simulink model "RotaryFlexLink_Workspace"  (R2021a)
settings: Solver=ode4  StartTime=0.0  StopTime=inf  FixedStep=0.001  RelTol=1e-3  EnableMultiTasking=on
model workspace (MAT data in the model file):
  Fc_est = 0.030885
  Jeq_est = 0.00174469
  Jl = 0.0038056
  Ll = 0.4191
  Rm_est = 3.11197
  beq_est = 0.0024798
  bl_est = 0.005635968
  km_est = 0.00744539
  ks_est = 1.3933
  kt_est = 0.00744539
  ml = 0.065
libraries: quarc_library x4, simulink x1
settings Model: SimulationMode=external  ExtModeTrigDuration=10000  Creator=MLevis  LastModifiedBy=pmartin
settings SolverCC: AlgebraicLoopSolver=TrustRegion  PositivePriorityOrder=on
settings DataIOCC: ReturnWorkspaceOutputs=off
settings DebuggingCC: SFMachineParentedDataDiag=warning  ArithmeticOperatorsInVariantConditions=warning
settings SFSimCC: SimUseLocalCustomCode=off  CustomCodeUndefinedFunction=UseInterfaceOnly
settings RTWCC: Description=QUARC Win64 Target Using Toolchain  SystemTargetFile=quarc_win64.tlc  TemplateMakefile=quarc_default_tmf  RTWUseLocalCustomCode=off  Toolchain=QUARC win64 | nmake (64-bit Windows)  BuildConfiguration=Faster Runs
settings CodeAppCC: StateflowObjectComments=on
settings STFCustomTargetCC: TargetLangStandard=C99 (ISO)  ConcurrentExecutionCompliant=on  SystemTargetFile=quarc_win64.tlc
settings GRTTargetCC: ParMdlRefBuildCompliant=off  CompOptLevelCompliant=off  CombineOutputUpdateFcns=off  MatFileLogging=off  CPPClassGenCompliant=off  GRTInterface=on  ExtMode=on  ExtModeMexFile=quarc_comm
settings ConfigComp: CovMetricSettings=dswe

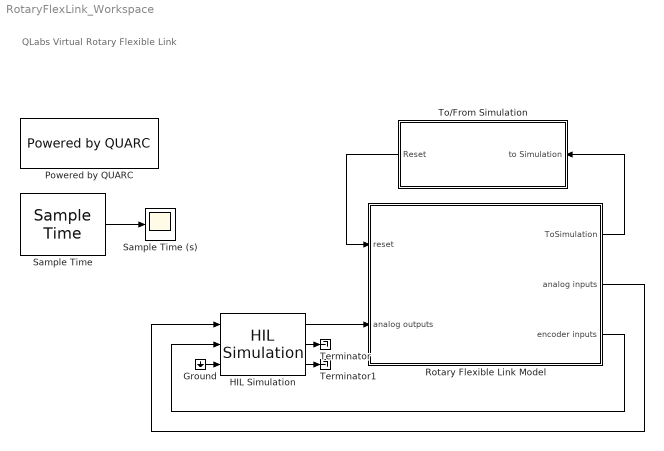
== system RotaryFlexLink_Workspace ==
  note: QLabs Virtual Rotary Flexible Link
  Ground : Ground
  HIL Simulation : quarc_library/Data Acquisition/Generic/Configuration/HIL Simulation  uri=tcpip://localhost:18941  board_type=q8_usb  board_id=0  sample_time=qc_get_step_size  active=on  num_clocks=1  num_interrupts=0  num_analog_inputs=8  num_analog_outputs=8  initial_analog=[]  num_digital_io=0  num_digital_inputs=8  num_digital_outputs=8  initial_digital=[]  num_encoder_inputs=8  num_pwm_outputs=8  initial_pwm=[]  other_inputs=[]  other_outputs=[]  initial_other=[]  integer_properties=[]  double_properties=[]  string_properties=[]
      settings: SourceProductName=QUARC Targets
  Powered by QUARC : quarc_library/Logos/Powered by QUARC
  Rotary Flexible Link Model : Subsystem
  Sample Time : quarc_library/Sources/Time/Sample Time  Priority=-99  sample_time=qc_get_step_size
  Sample Time (s) : Scope
  Terminator : Terminator
  Terminator1 : Terminator
  To/From Simulation : Subsystem
  wires:
  Rotary Flexible Link Model/3(encoder inputs) -> HIL Simulation/2
  Rotary Flexible Link Model/2(analog inputs) -> HIL Simulation/1
  HIL Simulation/1 -> Rotary Flexible Link Model/2(analog outputs)
  Sample Time/1 -> Sample Time (s)/1
  Rotary Flexible Link Model/1(ToSimulation) -> To/From Simulation/1(to Simulation)
  To/From Simulation/1(Reset) -> Rotary Flexible Link Model/1(reset)
  Ground/1 -> HIL Simulation/3
  HIL Simulation/2 -> Terminator/1
  HIL Simulation/3 -> Terminator1/1

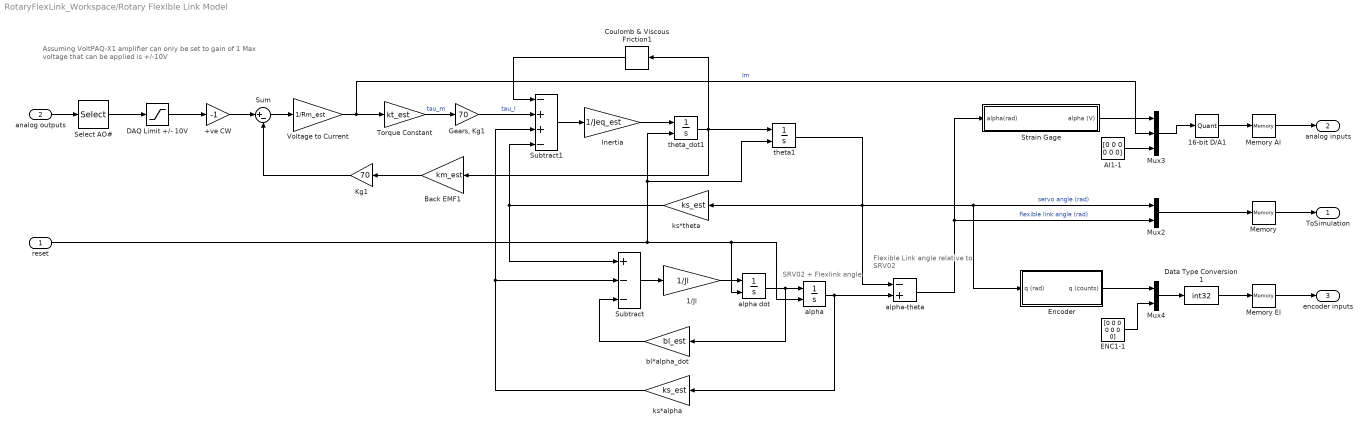
== system RotaryFlexLink_Workspace/Rotary Flexible Link Model ==
  note: Flexible Link angle
      | relative to SRV02
  note: SRV02 + Flexlink angle
  note: Assuming VoltPAQ-X1 amplifier can only be set to gain of 1
      | Max voltage that can be applied is +/-10V
  reset : Inport
  analog outputs : Inport  Port=2
  +ve CW : Gain  Gain=-1
  1/Jl : Gain  Gain=1/Jl  SaturateOnIntegerOverflow=on  OutDataTypeStr=Inherit: Same as input  ParamDataTypeStr=Inherit: Same as input
  16-bit D/A1 : Quantizer  QuantizationInterval=1/2^16
  AI1-1 : Constant  Value=[0 0 0 0 0 0]
  Back EMF1 : Gain  Gain=km_est  SaturateOnIntegerOverflow=on  OutDataTypeStr=Inherit: Same as input  ParamDataTypeStr=Inherit: Same as input
  Coulomb & Viscous Friction1 : simulink/Discontinuities/Coulomb & Viscous Friction  offset=[Fc_est]  gain=beq_est
  DAQ Limit +/- 10V : Saturate  UpperLimit=10  LowerLimit=-10
  Data Type Conversion1 : DataTypeConversion  OutDataTypeStr=int32
  ENC1-1 : Constant  Value=[0 0 0 0 0 0 0]
  Encoder : Subsystem
  "Gears, Kg1" : Gain  Gain=70
  Inertia : Gain  Gain=1/Jeq_est  SaturateOnIntegerOverflow=on  OutDataTypeStr=Inherit: Same as input  ParamDataTypeStr=Inherit: Same as input
  Kg1 : Gain  Gain=70
  Memory : Memory  InitialCondition=[0 0]
  Memory AI : Memory  InitialCondition=[0 0 0 0 0 0 0 0]  InheritSampleTime=on
  Memory EI : Memory  InitialCondition=[0 0 0 0 0 0 0 0]  InheritSampleTime=on
  Mux2 : Mux  Inputs=2
  Mux3 : Mux  Inputs=3
  Mux4 : Mux  Inputs=2
  Select AO# : Selector  InputPortWidth=8  IndexOptions=Index vector (dialog)  Indices=[1]  OutputSizes=1
  Strain Gage : Subsystem
  Subtract : Sum  Inputs=+--
  Subtract1 : Sum  Inputs=-++-
  Sum : Sum  Inputs=|+-  InputSameDT=on  SaturateOnIntegerOverflow=on  OutDataTypeStr=Inherit: Same as first input
  Torque Constant : Gain  Gain=kt_est
  Voltage to Current : Gain  Gain=1/Rm_est  SaturateOnIntegerOverflow=on  OutDataTypeStr=Inherit: Same as input  ParamDataTypeStr=Inherit: Same as input
  alpha : Integrator  ExternalReset=rising
  alpha dot : Integrator  ExternalReset=rising
  alpha-theta : Sum  Inputs=-+
  bl*alpha_dot : Gain  Gain=bl_est
  ks*alpha : Gain  Gain=ks_est
  ks*theta : Gain  Gain=ks_est
  theta1 : Integrator  ExternalReset=rising
  theta_dot1 : Integrator  ExternalReset=rising
  ToSimulation : Outport  VectorParamsAs1DForOutWhenUnconnected=off
  analog inputs : Outport  Port=2  VectorParamsAs1DForOutWhenUnconnected=off
  encoder inputs : Outport  Port=3  VectorParamsAs1DForOutWhenUnconnected=off
  wires:
  Memory/1 -> ToSimulation/1
  reset/1 -> theta1/2, theta_dot1/2, alpha dot/2, alpha/2
  Mux2/1 -> Memory/1
  Coulomb & Viscous Friction1/1 -> Subtract1/1
  Inertia/1 -> theta_dot1/1
  Sum/1 -> Voltage to Current/1
  bl*alpha_dot/1 -> Subtract/3
  ks*alpha/1 -> Subtract/2, Subtract1/3
  theta1/1 -> ks*theta/1, alpha-theta/1, Encoder/1(q (rad)), Mux2/1  "servo angle (rad)"
  Voltage to Current/1 -> Mux3/2, Torque Constant/1  "Im"
  Torque Constant/1 -> "Gears, Kg1"/1  "tau_m"
  Subtract/1 -> 1/Jl/1
  1/Jl/1 -> alpha dot/1
  Kg1/1 -> Sum/2
  ks*theta/1 -> Subtract/1, Subtract1/4
  "Gears, Kg1"/1 -> Subtract1/2  "tau_l"
  alpha dot/1 -> bl*alpha_dot/1, alpha/1
  theta_dot1/1 -> Coulomb & Viscous Friction1/1, theta1/1, Back EMF1/1
  Subtract1/1 -> Inertia/1
  alpha-theta/1 -> Strain Gage/1(alpha(rad)), Mux2/2  "flexible link angle (rad)"
  Back EMF1/1 -> Kg1/1
  +ve CW/1 -> Sum/1
  alpha/1 -> alpha-theta/2, ks*alpha/1
  analog outputs/1 -> Select AO#/1
  Select AO#/1 -> DAQ Limit +/- 10V/1
  DAQ Limit +/- 10V/1 -> +ve CW/1
  Mux3/1 -> 16-bit D/A1/1
  Encoder/1(q (counts)) -> Mux4/1
  Memory EI/1 -> encoder inputs/1
  Data Type Conversion1/1 -> Memory EI/1
  16-bit D/A1/1 -> Memory AI/1
  Mux4/1 -> Data Type Conversion1/1
  ENC1-1/1 -> Mux4/2
  AI1-1/1 -> Mux3/3
  Memory AI/1 -> analog inputs/1
  Strain Gage/1(alpha (V)) -> Mux3/1

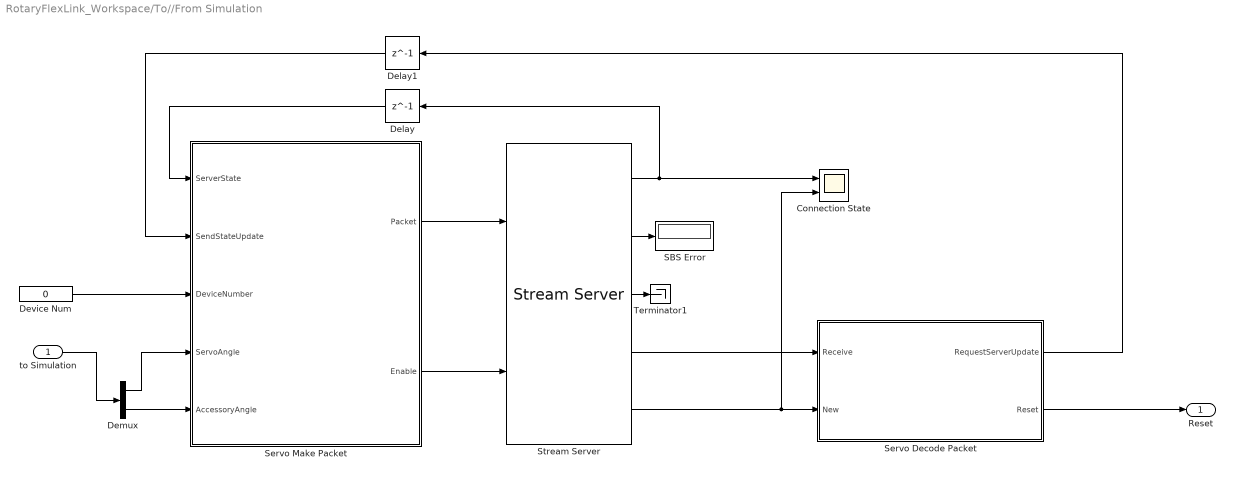
== system RotaryFlexLink_Workspace/To//From Simulation ==
  to Simulation : Inport
  "Connection State " : Scope  NumInputPorts=2
  Delay : Delay  DelayLength=1
  Delay1 : Delay  DelayLength=1
  Demux : Demux  Outputs=2
  Device Num : Constant  Value=0
  SBS Error : Display
  Servo Decode Packet : MATLAB Function  TreatAsAtomicUnit=on
  Servo Make Packet : MATLAB Function  TreatAsAtomicUnit=on
  Stream Server : quarc_library/Communications/Basic/Stream Server  uri_source=Specify via dialog (do not evaluate)  uri=tcpip://remotehost:18001?nagle='off'  apply_uri_to_all_configs=on  send_buffer_size=65537  receive_buffer_size=65537  byte_order=little endian (Intel - LSB first)  optimization=Minimum latency  send_options=Send all data  receive_options=Receive all data  default_value=[0]  sample_time=qc_get_step_size  active=on  implementation=Use blocking I/O in a separate thread  send_fifo_size=3  receive_fifo_size=3  send_priority=0  receive_priority=0  send_dimensions=on  receive_dimensions=on  max_dimensions=65537  data_type=uint8  type_expr=BusObject
      settings: AttributesFormatString="\"tcpip://remotehost:18001?nagle='off'\""
  Terminator1 : Terminator
  Reset : Outport  VectorParamsAs1DForOutWhenUnconnected=off
  wires:
  Stream Server/2 -> SBS Error/1
  Servo Decode Packet/2(Reset) -> Reset/1
  Stream Server/3 -> Terminator1/1
  Stream Server/1 -> Delay/1, "Connection State "/1
  Servo Make Packet/2(Enable) -> Stream Server/2
  Servo Decode Packet/1(RequestServerUpdate) -> Delay1/1
  Stream Server/5 -> "Connection State "/2, Servo Decode Packet/2(New)
  Servo Make Packet/1(Packet) -> Stream Server/1
  Stream Server/4 -> Servo Decode Packet/1(Receive)
  to Simulation/1 -> Demux/1
  Device Num/1 -> Servo Make Packet/3(DeviceNumber)
  Delay1/1 -> Servo Make Packet/2(SendStateUpdate)
  Delay/1 -> Servo Make Packet/1(ServerState)
  Demux/1 -> Servo Make Packet/4(ServoAngle)
  Demux/2 -> Servo Make Packet/5(AccessoryAngle)

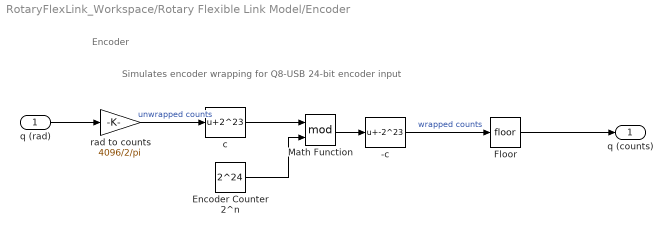
== system RotaryFlexLink_Workspace/Rotary Flexible Link Model/Encoder ==
  note: Encoder
  note: Simulates encoder wrapping for Q8-USB 24-bit encoder input
  q (rad) : Inport
  -c : Bias  Bias=-2^23
  Encoder Counter 2^n : Constant  Value=2^24
  Floor : Rounding
  Math Function : Math  Operator=mod  SignedPower=on  SaturateOnIntegerOverflow=on
  c : Bias  Bias=2^23
  rad to counts : Gain  Gain=4096/2/pi
  q (counts) : Outport  VectorParamsAs1DForOutWhenUnconnected=off
  wires:
  Math Function/1 -> -c/1
  q (rad)/1 -> rad to counts/1
  c/1 -> Math Function/1
  Encoder Counter 2^n/1 -> Math Function/2
  rad to counts/1 -> c/1  "unwrapped counts"
  -c/1 -> Floor/1  "wrapped counts"
  Floor/1 -> q (counts)/1

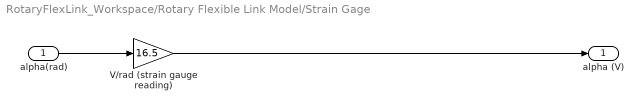
== system RotaryFlexLink_Workspace/Rotary Flexible Link Model/Strain Gage ==
  alpha(rad) : Inport
  V/rad (strain gauge reading) : Gain  Gain=16.5
  alpha (V) : Outport  VectorParamsAs1DForOutWhenUnconnected=off
  wires:
  alpha(rad)/1 -> V/rad (strain gauge reading)/1
  V/rad (strain gauge reading)/1 -> alpha (V)/1

== matlab function RotaryFlexLink_Workspace/To//From Simulation/Servo Make Packet ==
  settings: updateMethod=DISCRETE  sampleTime=qc_get_step_size
  data: Packet output size=65537; ServerState input; SendStateUpdate input; Enable output; DeviceNumber input; ServoAngle input; AccessoryAngle input
function [Packet,Enable] = RotaryFlexLinkMakePacket(ServerState, SendStateUpdate, DeviceNumber, ServoAngle, AccessoryAngle) 

% Be sure to set the maximum signal size of the variable size Packet port 
% in Simulink->Edit Data of the editor window.  Size should be 65537 or
% larger to ensure that the stream server generates a 4 byte packet size.

%% Setup
persistent LastServerState;

if isempty(LastServerState)
    LastServerState = uint8(0);
end

Enable = 0;
Packet = uint8([]);

%% On connection
if ((ServerState == 2) && (LastServerState ~= 2))
    Packet = RotaryFlexLinkMakeCommandStateContainer(DeviceNumber, ServoAngle, AccessoryAngle); 
end

%% Send new State Container
% Previous state processed, send a new one
if (SendStateUpdate)
    Packet = RotaryFlexLinkMakeCommandStateContainer(DeviceNumber, ServoAngle, AccessoryAngle); 
end

%% Transmit
% If we have data to send, enable the transmit
PacketLength = length(Packet);

if (PacketLength > 0)
    % Add magic byte.  This is just for error handling and isn't typically
    % required in simulink, but useful in lower-level languages like Python
    Packet = [uint8(123); Packet];
    
    Enable = 1; 
end


LastServerState = ServerState;

== matlab function RotaryFlexLink_Workspace/To//From Simulation/Servo Decode Packet ==
  data: Receive input size=65537; RequestServerUpdate output; New input; Reset output
function [RequestServerUpdate, Reset] = RotaryFlexLinkDecodePacket(Receive, New)

%% Setup



% Need to assign outputs here even though they are reassigned at the end
% since matlab can't determine the signal widths
Reset = 0;
RequestServerUpdate = 0;

PacketSize = length(Receive);

% Packet > 0, new data, and magic number in first index
if ((PacketSize > 0) && (New == 1) && (Receive(1) == uint8(123)))
    
    %skip magic number
    Index = int32(2);
    
    while(Index <= PacketSize)
       
        %% Get container details
        ContainerSize = typecast(uint8(flip(Receive(Index:Index+3))), 'int32');
        DeviceID = typecast(uint8(flip(Receive(Index+4:Index+7))), 'int32');
        DeviceNum = typecast(uint8(flip(Receive(Index+8:Index+11))), 'int32');
        DeviceFunction = uint8(Receive(Index+12));
        PayloadStart = Index+13;
        PayloadEnd = Index+ContainerSize-1;
        
        %% Pass container to appropriate decoding function
        if (DeviceID == 41) %is this a flexgauge container?
            
            if (DeviceFunction == 11) %UE4 State Response
                RequestServerUpdate = 1;
            end
        
        elseif (DeviceID == 1001) %Simulink notification
            if (DeviceFunction == 200) %Reset button
                Reset = 1;
            end
        end
        
        
        
        %% Process next container if any data is left.
        Index = Index+ContainerSize;
    end


end
